simulink subsystem "in_plane_velocity_direction"  (R2021b)
settings: Solver=VariableStepAuto  StartTime=0.0  StopTime=10.0  RelTol=1e-3
settings Model: Creator=austm  LastModifiedBy=austm

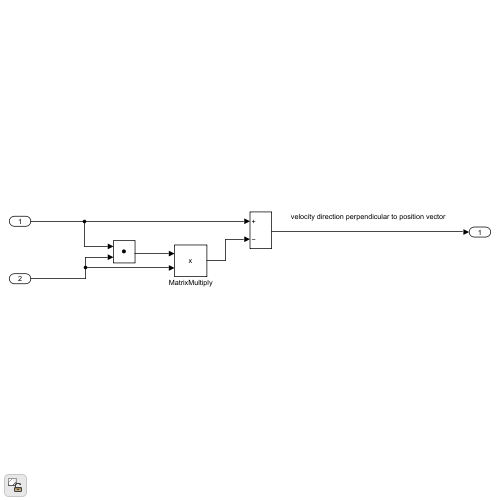
[thumbnail: Simulink's stored preview of the top-level diagram]
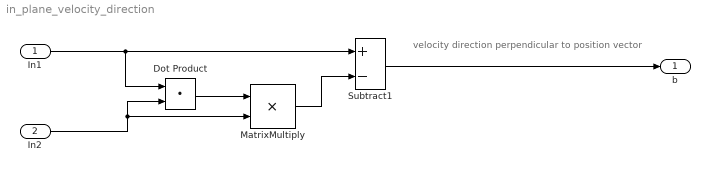
== system in_plane_velocity_direction ==
  note: velocity direction perpendicular to position vector
  In1 : Inport
  In2 : Inport  Port=2
  Dot Product : DotProduct  InputSameDT=on  OutDataTypeStr=Inherit: Inherit via internal rule
  MatrixMultiply : Product
  Subtract1 : Sum  Inputs=+-
  b : Outport
  wires:
  In1/1 -> Subtract1/1, Dot Product/1
  MatrixMultiply/1 -> Subtract1/2
  In2/1 -> MatrixMultiply/2, Dot Product/2
  Dot Product/1 -> MatrixMultiply/1
  Subtract1/1 -> b/1
